simulink model "untitled1"  (R2023b)
settings: Solver=FixedStepAuto  StartTime=0.0  StopTime=100  FixedStep=parameters.ts  RelTol=1e-3
undefined symbols (not defined in the file or in its folder): parameters
settings Model: Creator=death  LastModifiedBy=death
settings SolverCC: ZeroCrossAlgorithm=Adaptive
settings DebuggingCC: IgnoredZcDiagnostic=none

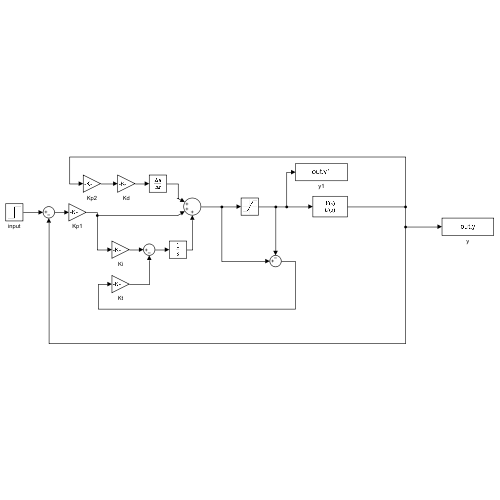
[thumbnail: Simulink's stored preview of the top-level diagram]
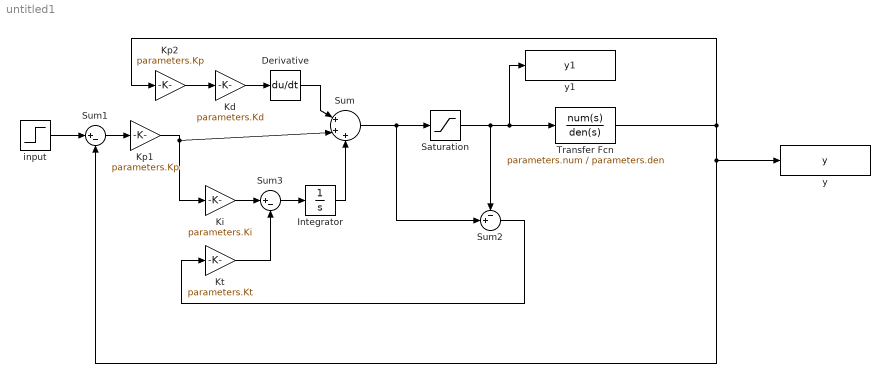
== system untitled1 ==
  Derivative : Derivative
  Integrator : Integrator
  Kd : Gain  Gain=parameters.Kd
  Ki : Gain  Gain=parameters.Ki
  Kp1 : Gain  Gain=parameters.Kp
  Kp2 : Gain  Gain=parameters.Kp
  Kt : Gain  Gain=parameters.Kt
  Saturation : Saturate  UpperLimit=parameters.upper_limit  LowerLimit=parameters.lower_limit
  Sum : Sum  Inputs=|+++
  Sum1 : Sum  Inputs=|+-
  Sum2 : Sum  Inputs=-+|
  Sum3 : Sum  Inputs=|+-
  Transfer Fcn : TransferFcn  Numerator=parameters.num  Denominator=parameters.den
  input : Step  Time=parameters.step_time  Before=parameters.initial_value  After=parameters.final_value  SampleTime=parameters.sample_time
  y : ToWorkspace  VariableName=y  SaveFormat=Structure With Time  SampleTime=0.5
  y1 : ToWorkspace  VariableName=y1  SaveFormat=Structure With Time  SampleTime=0.5
  wires:
  Transfer Fcn/1 -> Kp2/1, y/1, Sum1/2
  Integrator/1 -> Sum/3
  Sum/1 -> Sum2/2, Saturation/1
  Kp1/1 -> Sum/2, Ki/1
  input/1 -> Sum1/1
  Sum1/1 -> Kp1/1
  Ki/1 -> Sum3/1
  Sum3/1 -> Integrator/1
  Kt/1 -> Sum3/2
  Sum2/1 -> Kt/1
  Saturation/1 -> Transfer Fcn/1, y1/1, Sum2/1
  Kp2/1 -> Kd/1
  Kd/1 -> Derivative/1
  Derivative/1 -> Sum/1
